simulink model "PIUIO"  (R2016b)
settings: Solver=ode45  StartTime=0.0  StopTime=10.0  RelTol=1e-3  EnableMultiTasking=on
undefined symbols (not defined in the file): c1, d1Val, d2Val, d3Val, d4Val, d5Val, d6Val, d7Val, dist1, dist2, dist3, dist4, dist5, dist6, dist7, dt1, dt2, dt3, dt4, dt5, dt6, dt7, F, f1Val, f2Val, f3Val, f4Val, f5Val, f6Val, f7Val, flt1, flt2, flt3, flt4, flt5, flt6, flt7, G, J, L, M1, M2, n, N, tf1, tf2, tf3, tf4, tf5, tf6, tf7, x0
settings Model: Creator=sqn4594  LastModifiedBy=samnazari
settings DataIOCC: LimitDataPoints=on  SaveFormat=Array
settings OptimizationCC: LifeSpan=inf
settings DebuggingCC: SolverPrmCheckMsg=warning  FcnCallInpInsideContextMsg=warning  AllowSymbolicDim=off  SFUnexpectedBacktrackingDiag=warning  SFNoUnconditionalDefaultTransitionDiag=warning  SFExecutionAtInitializationDiag=none
settings HardwareCC: ProdBitPerPointer=32  ProdBitPerSizeT=32  ProdBitPerPtrDiffT=32  ProdLargestAtomicFloat=None  ProdIntDivRoundTo=Undefined  ProdEndianess=Unspecified  ProdWordSize=32  ProdHWDeviceType=32-bit Generic
settings ModelReferenceCC: PropagateSignalLabelsOutOfModel=off
settings GRTTargetCC: TargetLangStandard=C89/C90 (ANSI)  GeneratePreprocessorConditionals=Disable all
settings ConfigComp: CovMetricSettings=dw  CovHtmlReporting=on  CovSaveCumulativeToWorkspaceVar=on  CovSaveSingleToWorkspaceVar=on  CovExternalEMLEnable=off

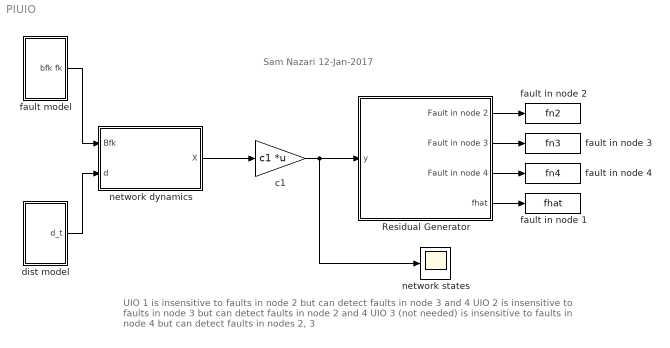
== system PIUIO ==
  note: UIO 1 is insensitive to faults in node 2 but can detect faults in node 3 and 4
      | UIO 2 is insensitive to faults in node 3 but can detect faults in node 2 and 4
      | UIO 3 (not needed) is insensitive to faults in node 4 but can detect faults in nodes 2, 3
  note: Sam Nazari
      | 12-Jan-2017
  Residual Generator : Subsystem
  c1 : Gain  Gain=c1  Multiplication=Matrix(K*u)
  dist model : Subsystem
  fault model : Subsystem
  fault in node 1 : ToWorkspace  VariableName=fhat  SaveFormat=Timeseries  SampleTime=-1
  fault in node 2 : ToWorkspace  VariableName=fn2  SaveFormat=Timeseries  SampleTime=-1
  fault in node 3 : ToWorkspace  VariableName=fn3  SaveFormat=Timeseries  SampleTime=-1
  fault in node 4 : ToWorkspace  VariableName=fn4  SaveFormat=Timeseries  SampleTime=-1
  network dynamics : Subsystem
  network states : Scope
  wires:
  fault model/1(bfk fk) -> network dynamics/1(Bfk)
  network dynamics/1(X) -> c1/1
  c1/1 -> network states/1, Residual Generator/1(y)
  dist model/1(d_t) -> network dynamics/2(d)
  Residual Generator/1(Fault in node 2) -> fault in node 2/1
  Residual Generator/2(Fault in node 3) -> fault in node 3/1
  Residual Generator/3(Fault in node 4) -> fault in node 4/1
  Residual Generator/4(fhat) -> fault in node 1/1

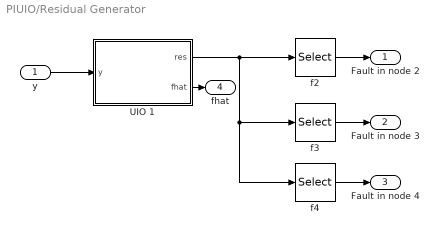
== system PIUIO/Residual Generator ==
  y : Inport
  UIO 1 : Subsystem
  f2 : Selector  InputPortWidth=3  IndexOptions=Index vector (dialog)  Indices=1  OutputSizes=1
  f3 : Selector  InputPortWidth=3  IndexOptions=Index vector (dialog)  Indices=2  OutputSizes=1
  f4 : Selector  InputPortWidth=3  IndexOptions=Index vector (dialog)  Indices=3  OutputSizes=1
  Fault in node 2 : Outport
  Fault in node 3 : Outport  Port=2
  Fault in node 4 : Outport  Port=3
  fhat : Outport  Port=4
  wires:
  y/1 -> UIO 1/1(y)
  f2/1 -> Fault in node 2/1
  f3/1 -> Fault in node 3/1
  UIO 1/1(res) -> f4/1, f3/1, f2/1
  f4/1 -> Fault in node 4/1
  UIO 1/2(fhat) -> fhat/1

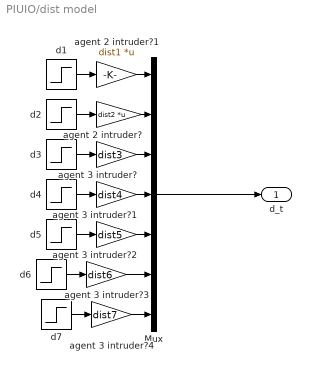
== system PIUIO/dist model ==
  Mux : Mux  Inputs=7
  agent 2 intruder? : Gain  Gain=dist2  Multiplication=Matrix(K*u)
  agent 2 intruder?1 : Gain  Gain=dist1  Multiplication=Matrix(K*u)
  agent 3 intruder? : Gain  Gain=dist3
  agent 3 intruder?1 : Gain  Gain=dist4
  agent 3 intruder?2 : Gain  Gain=dist5
  agent 3 intruder?3 : Gain  Gain=dist6
  agent 3 intruder?4 : Gain  Gain=dist7
  d1 : Step  After=d1Val  SampleTime=dt1
  d2 : Step  After=d2Val  SampleTime=dt2
  d3 : Step  After=d3Val  SampleTime=dt3
  d4 : Step  After=d4Val  SampleTime=dt4
  d5 : Step  After=d5Val  SampleTime=dt5
  d6 : Step  After=d6Val  SampleTime=dt6
  d7 : Step  After=d7Val  SampleTime=dt7
  d_t : Outport
  wires:
  Mux/1 -> d_t/1
  d1/1 -> agent 2 intruder?1/1
  d2/1 -> agent 2 intruder?/1
  d3/1 -> agent 3 intruder?/1
  agent 2 intruder?/1 -> Mux/2
  agent 3 intruder?/1 -> Mux/3
  agent 2 intruder?1/1 -> Mux/1
  d4/1 -> agent 3 intruder?1/1
  agent 3 intruder?1/1 -> Mux/4
  agent 3 intruder?2/1 -> Mux/5
  d5/1 -> agent 3 intruder?2/1
  d6/1 -> agent 3 intruder?3/1
  agent 3 intruder?3/1 -> Mux/6
  d7/1 -> agent 3 intruder?4/1
  agent 3 intruder?4/1 -> Mux/7

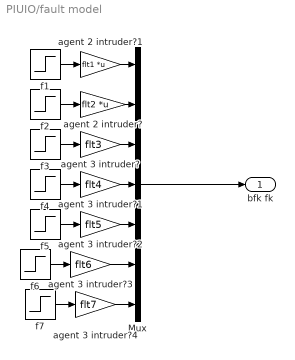
== system PIUIO/fault model ==
  Mux : Mux  Inputs=7
  agent 2 intruder? : Gain  Gain=flt2  Multiplication=Matrix(K*u)
  agent 2 intruder?1 : Gain  Gain=flt1  Multiplication=Matrix(K*u)
  agent 3 intruder? : Gain  Gain=flt3
  agent 3 intruder?1 : Gain  Gain=flt4
  agent 3 intruder?2 : Gain  Gain=flt5
  agent 3 intruder?3 : Gain  Gain=flt6
  agent 3 intruder?4 : Gain  Gain=flt7
  f1 : Step  After=f1Val  SampleTime=tf1
  f2 : Step  After=f2Val  SampleTime=tf2
  f3 : Step  After=f3Val  SampleTime=tf3
  f4 : Step  After=f4Val  SampleTime=tf4
  f5 : Step  After=f5Val  SampleTime=tf5
  f6 : Step  After=f6Val  SampleTime=tf6
  f7 : Step  After=f7Val  SampleTime=tf7
  bfk fk : Outport
  wires:
  Mux/1 -> bfk fk/1
  f1/1 -> agent 2 intruder?1/1
  f2/1 -> agent 2 intruder?/1
  f3/1 -> agent 3 intruder?/1
  agent 2 intruder?/1 -> Mux/2
  agent 3 intruder?/1 -> Mux/3
  agent 2 intruder?1/1 -> Mux/1
  f4/1 -> agent 3 intruder?1/1
  agent 3 intruder?1/1 -> Mux/4
  agent 3 intruder?2/1 -> Mux/5
  f5/1 -> agent 3 intruder?2/1
  f6/1 -> agent 3 intruder?3/1
  agent 3 intruder?3/1 -> Mux/6
  f7/1 -> agent 3 intruder?4/1
  agent 3 intruder?4/1 -> Mux/7

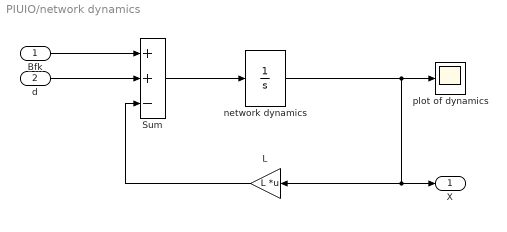
== system PIUIO/network dynamics ==
  Bfk : Inport
  d : Inport  Port=2
  L : Gain  Gain=L  Multiplication=Matrix(K*u)
  Sum : Sum  Inputs=++-
  network dynamics : Integrator  InitialCondition=x0
  plot of dynamics : Scope
  X : Outport
  wires:
  Sum/1 -> network dynamics/1
  network dynamics/1 -> plot of dynamics/1, X/1, L/1
  L/1 -> Sum/3
  Bfk/1 -> Sum/1
  d/1 -> Sum/2

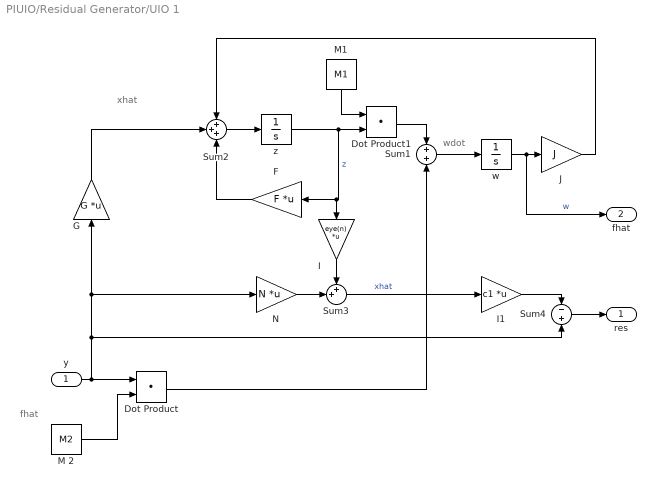
== system PIUIO/Residual Generator/UIO 1 ==
  note: xhat
  note: wdot
  note: fhat
  y : Inport
  Dot Product : DotProduct  InputSameDT=on  OutDataTypeStr=Inherit: Inherit via internal rule
  Dot Product1 : DotProduct  InputSameDT=on  OutDataTypeStr=Inherit: Inherit via internal rule
  F : Gain  Gain=F  Multiplication=Matrix(K*u)
  G : Gain  Gain=G  Multiplication=Matrix(K*u)
  I : Gain  Gain=eye(n)  Multiplication=Matrix(K*u)
  I1 : Gain  Gain=c1  Multiplication=Matrix(K*u)
  J : Gain  Gain=J
  M 2 : Constant  Value=M2
  "M1 " : Constant  Value=M1
  N : Gain  Gain=N  Multiplication=Matrix(K*u) (u vector)
  Sum1 : Sum
  Sum2 : Sum  Inputs=+++
  Sum3 : Sum  Inputs=++|
  Sum4 : Sum  Inputs=-+
  w : Integrator  InitialCondition=x0
  z : Integrator  InitialCondition=x0
  res : Outport
  fhat : Outport  Port=2
  wires:
  Sum2/1 -> z/1
  z/1 -> Dot Product1/2, F/1, I/1  "z"
  F/1 -> Sum2/3
  y/1 -> Dot Product/1, Sum4/2, N/1, G/1
  G/1 -> Sum2/2
  M 2/1 -> Dot Product/2
  Dot Product/1 -> Sum1/2
  Dot Product1/1 -> Sum1/1
  "M1 "/1 -> Dot Product1/1
  Sum1/1 -> w/1
  w/1 -> fhat/1, J/1  "w"
  J/1 -> Sum2/1
  I/1 -> Sum3/1
  N/1 -> Sum3/2
  Sum3/1 -> I1/1  "xhat"
  I1/1 -> Sum4/1
  Sum4/1 -> res/1
